simulink model "model_ciagly"  (Simulink 7.5)
settings: Solver=ode45  StartTime=0.0  StopTime=5  MaxStep=0.001  RelTol=1e-3
values from neighbouring files (symbols this model uses):
  Kp = 1.5*Un/10    [dane_sym.m]
  Kt = 10/1.5/wn    [dane_sym.m]
  wn = nn*2*pi/60    [dane_sym.m]
  Y = 10/2.5/In    [dane_sym.m]
undefined symbols (not defined in the file or in its folder): B, In, J, Kw, lambdaN, m, Mn, psien, Rt, T, tm, Tr, Un, uz0, V
settings Model: Creator=Konrad  LastModifiedBy=Konrad

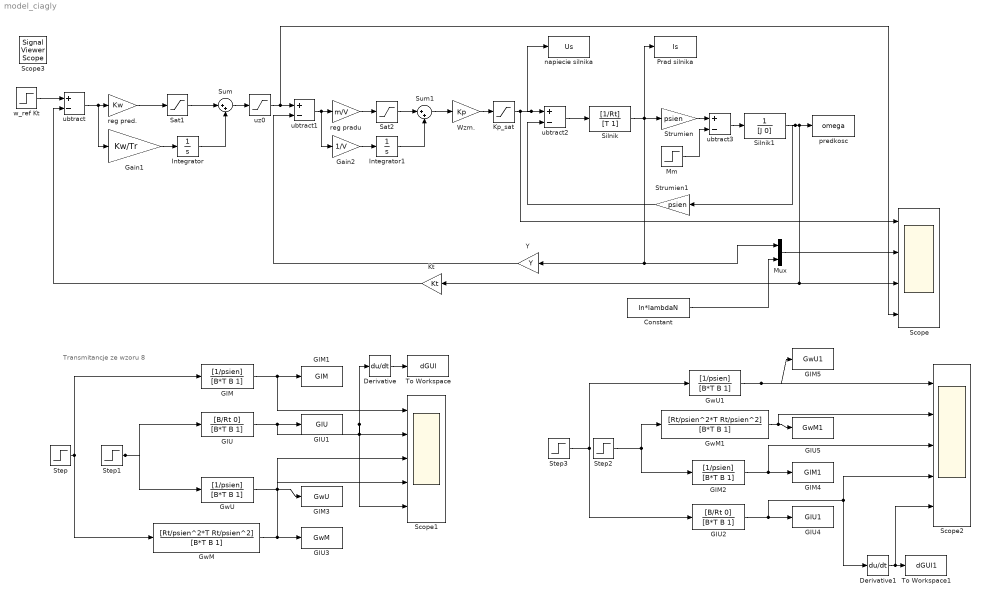
== system model_ciagly ==
  note: Transmitancje ze wzoru 8
  Constant : Constant  Value=In*lambdaN  OutDataType=fixdt(1, 16)  OutScaling=2^0
  Derivative : Derivative
  Derivative1 : Derivative
  GIM : TransferFcn  Numerator=[1/psien]  Denominator=[B*T B 1]
  GIM1 : ToWorkspace  VariableName=GIM  SampleTime=-1  SaveFormat=Structure With Time
  GIM2 : TransferFcn  Numerator=[1/psien]  Denominator=[B*T B 1]
  GIM3 : ToWorkspace  VariableName=GwU  SampleTime=-1  SaveFormat=Structure With Time
  GIM4 : ToWorkspace  VariableName=GIM1  SampleTime=-1  SaveFormat=Structure With Time
  GIM5 : ToWorkspace  VariableName=GwU1  SampleTime=-1  SaveFormat=Structure With Time
  GIU : TransferFcn  Numerator=[B/Rt 0]  Denominator=[B*T B 1]
  GIU1 : ToWorkspace  VariableName=GIU  SampleTime=-1  SaveFormat=Structure With Time
  GIU2 : TransferFcn  Numerator=[B/Rt 0]  Denominator=[B*T B 1]
  GIU3 : ToWorkspace  VariableName=GwM  SampleTime=-1  SaveFormat=Structure With Time
  GIU4 : ToWorkspace  VariableName=GIU1  SampleTime=-1  SaveFormat=Structure With Time
  GIU5 : ToWorkspace  VariableName=GwM1  SampleTime=-1  SaveFormat=Structure With Time
  Gain1 : Gain  Gain=Kw/Tr  ParameterDataType=fixdt(1, 16)  ParameterScaling=2^0  OutDataType=fixdt(1, 16)  OutScaling=2^0
  Gain2 : Gain  Gain=1/V  ParameterDataType=fixdt(1, 16)  ParameterScaling=2^0  OutDataType=fixdt(1, 16)  OutScaling=2^0
  GwM : TransferFcn  Numerator=[Rt/psien^2*T Rt/psien^2]  Denominator=[B*T B 1]
  GwM1 : TransferFcn  Numerator=[Rt/psien^2*T Rt/psien^2]  Denominator=[B*T B 1]
  GwU : TransferFcn  Numerator=[1/psien]  Denominator=[B*T B 1]
  GwU1 : TransferFcn  Numerator=[1/psien]  Denominator=[B*T B 1]
  Integrator : Integrator  LimitOutput=on  UpperSaturationLimit=10  LowerSaturationLimit=-10
  Integrator1 : Integrator  LimitOutput=on  UpperSaturationLimit=10  LowerSaturationLimit=-10
  Kp_sat : Saturate  UpperLimit=1.5*Un  LowerLimit=-1.5*Un  OutDataType=fixdt(1, 16)  OutScaling=2^0
  Kt : Gain  Gain=Kt  ParameterDataType=fixdt(1, 16)  ParameterScaling=2^0  OutDataType=fixdt(1, 16)  OutScaling=2^0
  Mm : Step  Time=tm  After=Mn  SampleTime=0
  Mux : Mux  Inputs=2
  Prad silnika : ToWorkspace  VariableName=Is  SampleTime=-1  SaveFormat=Structure
  Sat1 : Saturate  UpperLimit=10  LowerLimit=-10  OutDataType=fixdt(1, 16)  OutScaling=2^0
  Sat2 : Saturate  UpperLimit=10  LowerLimit=-10  OutDataType=fixdt(1, 16)  OutScaling=2^0
  Scope : Scope  NumInputPorts=4
      settings: YMin=-5~-5~-5~-5  YMax=5~5~5~5
  Scope1 : Scope  NumInputPorts=5
      settings: YMin=-5~-5~-5~-5~-5  YMax=5~5~5~5~5
  Scope2 : Scope  NumInputPorts=5
      settings: YMin=-5~-5~-5~-5~-5  YMax=5~5~5~5~5  SaveName=ScopeData2
  Silnik : TransferFcn  Numerator=[1/Rt]  Denominator=[T 1]
  Silnik1 : TransferFcn  Denominator=[J 0]
  Step : Step  After=psien*In  SampleTime=0
  Step1 : Step  After=Un  SampleTime=0
  Step2 : Step  After=psien*In  SampleTime=0
  Step3 : Step  After=Un  SampleTime=0
  Strumien : Gain  Gain=psien  ParameterDataType=fixdt(1, 16)  ParameterScaling=2^0  OutDataType=fixdt(1, 16)  OutScaling=2^0
  Strumien1 : Gain  Gain=psien  ParameterDataType=fixdt(1, 16)  ParameterScaling=2^0  OutDataType=fixdt(1, 16)  OutScaling=2^0
  Sum : Sum  Inputs=|++  OutDataType=fixdt(1, 16)  OutScaling=2^0
  Sum1 : Sum  Inputs=|++  OutDataType=fixdt(1, 16)  OutScaling=2^0
  To Workspace : ToWorkspace  VariableName=dGUI  SampleTime=-1  SaveFormat=Structure
  To Workspace1 : ToWorkspace  VariableName=dGUI1  SampleTime=-1  SaveFormat=Structure
  Wzm. : Gain  Gain=Kp  ParameterDataType=fixdt(1, 16)  ParameterScaling=2^0  OutDataType=fixdt(1, 16)  OutScaling=2^0
  Y : Gain  Gain=Y  ParameterDataType=fixdt(1, 16)  ParameterScaling=2^0  OutDataType=fixdt(1, 16)  OutScaling=2^0
  napiecie silnika : ToWorkspace  VariableName=Us  SampleTime=-1  SaveFormat=Structure
  predkosc : ToWorkspace  VariableName=omega  SampleTime=-1  SaveFormat=Structure
  reg pradu : Gain  Gain=m/V  ParameterDataType=fixdt(1, 16)  ParameterScaling=2^0  OutDataType=fixdt(1, 16)  OutScaling=2^0
  reg pred. : Gain  Gain=Kw  ParameterDataType=fixdt(1, 16)  ParameterScaling=2^0  OutDataType=fixdt(1, 16)  OutScaling=2^0
  ubtract{,1..3} (4 alike) : Sum  Inputs=+-  OutDataType=fixdt(1, 16)  OutScaling=2^-10
  uz0 : Saturate  UpperLimit=uz0  LowerLimit=-uz0  OutDataType=fixdt(1, 16)  OutScaling=2^0
  w_ref Kt : Step  Time=0  After=wn*Kt  SampleTime=0
  Scope3 : SignalViewerScope  IOType=viewer  RefreshTime=0.035000
      settings: ShowLegends=on
  wires:
  w_ref Kt/1 -> ubtract/1
  ubtract/1 -> reg pred./1, Gain1/1
  reg pred./1 -> Sat1/1
  Sat1/1 -> Sum/1
  Gain1/1 -> Integrator/1
  Integrator/1 -> Sum/2
  Sum/1 -> uz0/1
  uz0/1 -> ubtract1/1, Scope/4
  ubtract1/1 -> reg pradu/1, Gain2/1
  reg pradu/1 -> Sat2/1
  Sat2/1 -> Sum1/1
  Gain2/1 -> Integrator1/1
  Integrator1/1 -> Sum1/2
  Sum1/1 -> Wzm./1
  Wzm./1 -> Kp_sat/1
  Kp_sat/1 -> ubtract2/1, napiecie silnika/1, Scope/1
  ubtract2/1 -> Silnik/1
  Silnik/1 -> Strumien/1, Prad silnika/1, Mux/1, Y/1
  Strumien/1 -> ubtract3/1
  Mm/1 -> ubtract3/2
  ubtract3/1 -> Silnik1/1
  Silnik1/1 -> Strumien1/1, predkosc/1, Scope/3, Kt/1
  Mux/1 -> Scope/2
  Strumien1/1 -> ubtract2/2
  Y/1 -> ubtract1/2
  Kt/1 -> ubtract/2
  Constant/1 -> Mux/2
  GIM/1 -> Scope1/1, GIM1/1
  GIU/1 -> GIU1/1, Scope1/2, Derivative/1, Scope1/5
  Step1/1 -> GIU/1, GwU/1
  Step/1 -> GIM/1, GwM/1
  GwU/1 -> GIM3/1, Scope1/3
  GwM/1 -> GIU3/1, Scope1/4
  Derivative/1 -> To Workspace/1
  Derivative1/1 -> To Workspace1/1, Scope2/5
  GwU1/1 -> GIM5/1, Scope2/1
  GwM1/1 -> GIU5/1, Scope2/2
  GIM2/1 -> GIM4/1, Scope2/3
  GIU2/1 -> GIU4/1, Scope2/4, Derivative1/1
  Step2/1 -> GwM1/1, GIM2/1
  Step3/1 -> GwU1/1, GIU2/1
